simulink library "motorLibrary"  (R2020b)
settings: Solver=VariableStepAuto  StartTime=0.0  StopTime=10.0  RelTol=1e-3
undefined symbols (not defined in the file): convert, motor
settings Model: Creator=ericb  LastModifiedBy=ericb

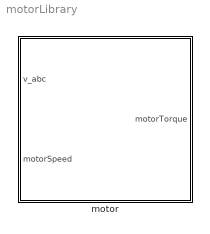
== system motorLibrary ==
  motor : Subsystem  Variant=on

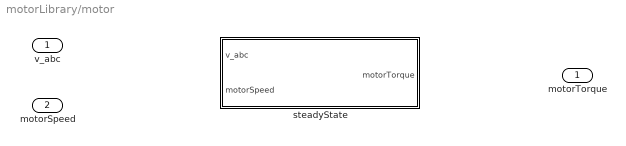
== system motorLibrary/motor ==
  v_abc : Inport
  motorSpeed : Inport  Port=2
  steadyState : Subsystem  VariantControl=strcmp(motor.blockChoice,'steadyState')
  motorTorque : Outport

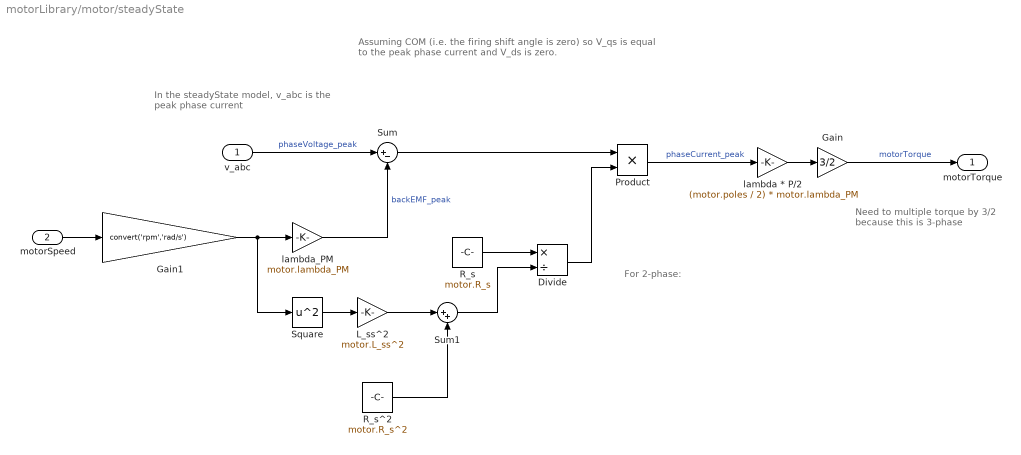
== system motorLibrary/motor/steadyState ==
  note: Need to multiple torque by 3/2 because this is 3-phase
  note: For 2-phase:
  note: Assuming COM (i.e. the firing shift angle is zero) so V_qs is equal to the peak phase current and V_ds is zero.
  note: In the steadyState model, v_abc is the peak phase current
  v_abc : Inport
  motorSpeed : Inport  Port=2
  Divide : Product  Inputs=*/
  Gain : Gain  Gain=3/2
  Gain1 : Gain  Gain=convert('rpm','rad/s')
  L_ss^2 : Gain  Gain=motor.L_ss^2
  Product : Product
  R_s : Constant  Value=motor.R_s
  R_s^2 : Constant  Value=motor.R_s^2
  Square : Math  Operator=square  SaturateOnIntegerOverflow=on
  Sum : Sum  Inputs=|+-
  Sum1 : Sum  Inputs=|++
  lambda * P/2 : Gain  Gain=(motor.poles / 2) * motor.lambda_PM
  lambda_PM : Gain  Gain=motor.lambda_PM
  motorTorque : Outport
  wires:
  motorSpeed/1 -> Gain1/1
  v_abc/1 -> Sum/1  "phaseVoltage_peak"
  lambda_PM/1 -> Sum/2  "backEMF_peak"
  Gain/1 -> motorTorque/1  "motorTorque"
  Square/1 -> L_ss^2/1
  L_ss^2/1 -> Sum1/1
  R_s^2/1 -> Sum1/2
  Sum1/1 -> Divide/2
  R_s/1 -> Divide/1
  Sum/1 -> Product/1
  Divide/1 -> Product/2
  Product/1 -> lambda * P/2/1  "phaseCurrent_peak"
  lambda * P/2/1 -> Gain/1
  Gain1/1 -> Square/1, lambda_PM/1
